simulink model "lateral_control"  (Simulink 7.6)
settings: Solver=FixedStepDiscrete  StartTime=0.0  StopTime=Tfin  FixedStep=Ts  RelTol=1e-3
undefined symbols (not defined in the file or in its folder): ailerons_max, ailerons_min, ailerons_trim, beta_trim, DiscIntNeverNeededParam, K_heading, K_roll, roll_trim, rollrate_trim, rudder_max, rudder_trim, yawrate_trim
libraries: simulink x2
settings Model: Creator=borjafons  LastModifiedBy=frafonal
settings OptimizationCC: InlineParams=on  OptimizeModelRefInitCode=on  LifeSpan=1
settings DebuggingCC: FcnCallInpInsideContextMsg=Enable All
settings RTWCC: SystemTargetFile=ert.tlc  GenCodeOnly=on  TemplateMakefile=ert_default_tmf  Description=Embedded Coder  ProcessScript=ert_make_rtw_hook
settings CodeAppCC: IgnoreCustomStorageClasses=off
settings ERTTargetCC: MultiwordLength=2048  GenerateSampleERTMain=on  SupportNonFinite=off  SupportComplex=off  InlinedParameterPlacement=NonHierarchical  ERTCustomFileTemplate=example_file_process.tlc  ConvertIfToSwitch=off

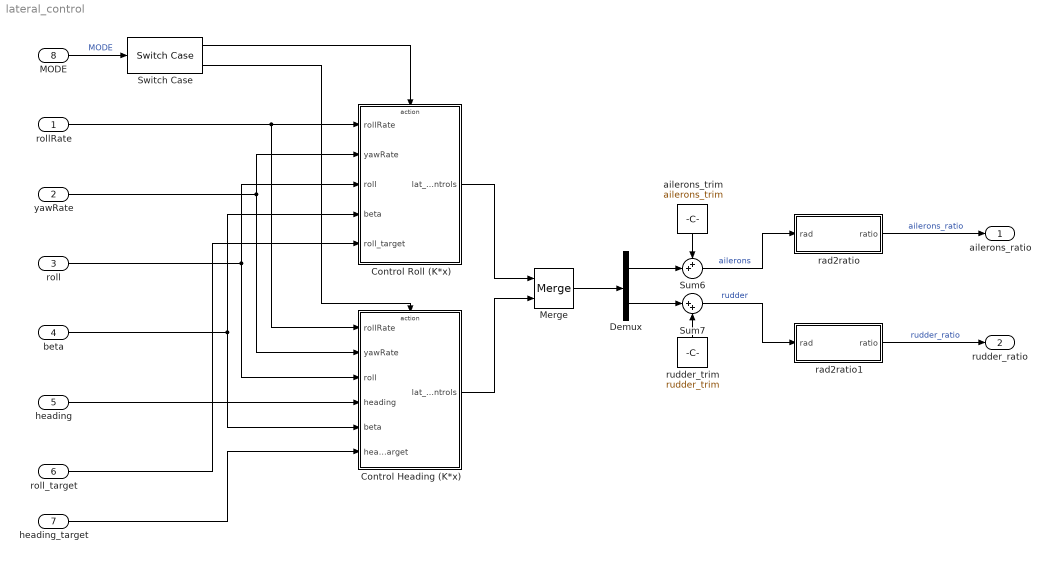
== system lateral_control ==
  rollRate : Inport
  yawRate : Inport  Port=2
  roll : Inport  Port=3
  beta : Inport  Port=4
  heading : Inport  Port=5
  roll_target : Inport  Port=6
  heading_target : Inport  Port=7
  MODE : Inport  Port=8
  Control Heading (K*x) : Subsystem  TreatAsAtomicUnit=on
  Control Roll (K*x) : Subsystem  TreatAsAtomicUnit=on
  Demux : Demux  Outputs=2
  Merge : Merge
  Sum6 : Sum  Inputs=++|
  Sum7 : Sum  Inputs=|++
  Switch Case : SwitchCase  CaseConditions={ROLL_CONTROL, HEADING_CONTROL}  ShowDefaultCase=off
  ailerons_trim : Constant  Value=ailerons_trim
  rad2ratio : Subsystem
  rad2ratio1 : Subsystem
  rudder_trim : Constant  Value=rudder_trim
  ailerons_ratio : Outport
  rudder_ratio : Outport  Port=2
  wires:
  Merge/1 -> Demux/1
  rad2ratio/1(ratio) -> ailerons_ratio/1  "ailerons_ratio"
  rad2ratio1/1(ratio) -> rudder_ratio/1  "rudder_ratio"
  ailerons_trim/1 -> Sum6/1
  Sum6/1 -> rad2ratio/1(rad)  "ailerons"
  Demux/1 -> Sum6/2
  rudder_trim/1 -> Sum7/2
  Demux/2 -> Sum7/1
  Sum7/1 -> rad2ratio1/1(rad)  "rudder"
  Control Roll (K*x)/1(lat_controls) -> Merge/1
  Control Heading (K*x)/1(lat_controls) -> Merge/2
  Switch Case/1 -> Control Roll (K*x)/Action
  MODE/1 -> Switch Case/1  "MODE"
  rollRate/1 -> Control Roll (K*x)/1(rollRate), Control Heading (K*x)/1(rollRate)
  yawRate/1 -> Control Roll (K*x)/2(yawRate), Control Heading (K*x)/2(yawRate)
  roll/1 -> Control Roll (K*x)/3(roll), Control Heading (K*x)/3(roll)
  beta/1 -> Control Roll (K*x)/4(beta), Control Heading (K*x)/5(beta)
  heading/1 -> Control Heading (K*x)/4(heading)
  roll_target/1 -> Control Roll (K*x)/5(roll_target)
  heading_target/1 -> Control Heading (K*x)/6(heading_target)
  Switch Case/2 -> Control Heading (K*x)/Action

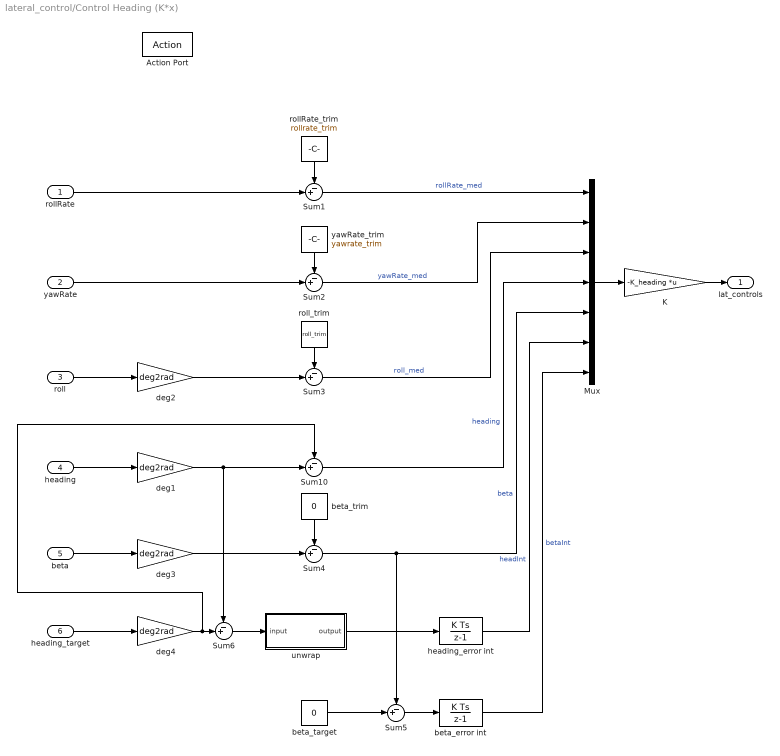
== system lateral_control/Control Heading (K*x) ==
  rollRate : Inport
  yawRate : Inport  Port=2
  roll : Inport  Port=3
  heading : Inport  Port=4
  beta : Inport  Port=5
  heading_target : Inport  Port=6
  Action Port : ActionPort  ActionType=case
  K : Gain  Gain=-K_heading  Multiplication=Matrix(K*u) (u vector)
  Mux : Mux  Inputs=7
  Sum{1..6,10} (7 alike) : Sum  Inputs=-+|
  beta_error int : DiscreteIntegrator  SampleTime=-1  LimitOutput=on  UpperSaturationLimit=5  LowerSaturationLimit=-5  ICPrevOutput=DiscIntNeverNeededParam  ICPrevScaledInput=DiscIntNeverNeededParam
  beta_target : Constant  Value=0
  beta_trim : Constant  Value=0
  deg{1..4} (4 alike) : Gain  Gain=deg2rad
  heading_error int : DiscreteIntegrator  SampleTime=-1  LimitOutput=on  UpperSaturationLimit=20  LowerSaturationLimit=-20  ICPrevOutput=DiscIntNeverNeededParam  ICPrevScaledInput=DiscIntNeverNeededParam
  rollRate_trim : Constant  Value=rollrate_trim
  roll_trim : Constant  Value=roll_trim
  unwrap : Subsystem
  yawRate_trim : Constant  Value=yawrate_trim
  lat_controls : Outport
  wires:
  Mux/1 -> K/1
  K/1 -> lat_controls/1
  rollRate_trim/1 -> Sum1/1
  rollRate/1 -> Sum1/2
  yawRate_trim/1 -> Sum2/1
  yawRate/1 -> Sum2/2
  roll_trim/1 -> Sum3/1
  roll/1 -> deg2/1
  deg2/1 -> Sum3/2
  Sum1/1 -> Mux/1  "rollRate_med"
  Sum2/1 -> Mux/2  "yawRate_med"
  Sum3/1 -> Mux/3  "roll_med"
  heading/1 -> deg1/1
  beta/1 -> deg3/1
  deg1/1 -> Sum10/2, Sum6/1
  beta_trim/1 -> Sum4/1
  deg3/1 -> Sum4/2
  Sum10/1 -> Mux/4  "heading"
  Sum4/1 -> Mux/5, Sum5/1  "beta"
  beta_target/1 -> Sum5/2
  Sum5/1 -> beta_error int/1
  beta_error int/1 -> Mux/7  "betaInt"
  heading_target/1 -> deg4/1
  deg4/1 -> Sum6/2, Sum10/1
  Sum6/1 -> unwrap/1(input)
  unwrap/1(output) -> heading_error int/1
  heading_error int/1 -> Mux/6  "headInt"

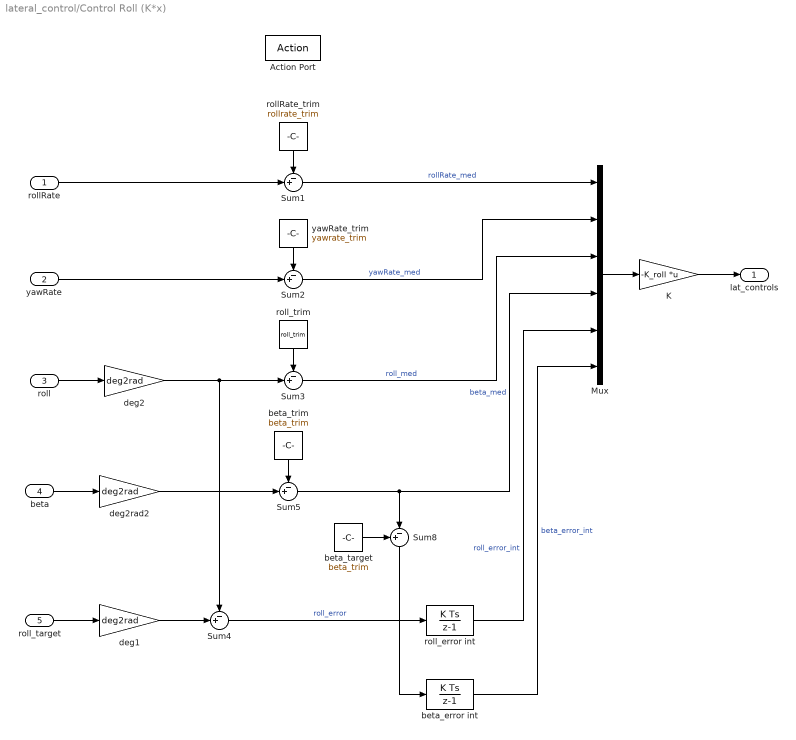
== system lateral_control/Control Roll (K*x) ==
  rollRate : Inport
  yawRate : Inport  Port=2
  roll : Inport  Port=3
  beta : Inport  Port=4
  roll_target : Inport  Port=5
  Action Port : ActionPort  ActionType=case
  K : Gain  Gain=-K_roll  Multiplication=Matrix(K*u) (u vector)
  Mux : Mux  Inputs=6
  Sum{1..5} (5 alike) : Sum  Inputs=-+|
  Sum8 : Sum  Inputs=+-|
  beta_error int : DiscreteIntegrator  SampleTime=-1  LimitOutput=on  UpperSaturationLimit=5  LowerSaturationLimit=-5  ICPrevOutput=DiscIntNeverNeededParam  ICPrevScaledInput=DiscIntNeverNeededParam
  beta_target : Constant  Value=beta_trim
  beta_trim : Constant  Value=beta_trim
  deg1 : Gain  Gain=deg2rad
  deg2 : Gain  Gain=deg2rad
  deg2rad2 : Gain  Gain=deg2rad
  rollRate_trim : Constant  Value=rollrate_trim
  roll_error int : DiscreteIntegrator  SampleTime=-1  LimitOutput=on  UpperSaturationLimit=8  LowerSaturationLimit=-8  ICPrevOutput=DiscIntNeverNeededParam  ICPrevScaledInput=DiscIntNeverNeededParam
  roll_trim : Constant  Value=roll_trim
  yawRate_trim : Constant  Value=yawrate_trim
  lat_controls : Outport
  wires:
  Mux/1 -> K/1
  K/1 -> lat_controls/1
  rollRate_trim/1 -> Sum1/1
  rollRate/1 -> Sum1/2
  yawRate_trim/1 -> Sum2/1
  yawRate/1 -> Sum2/2
  roll_trim/1 -> Sum3/1
  roll/1 -> deg2/1
  deg2/1 -> Sum3/2, Sum4/1
  beta_trim/1 -> Sum5/1
  deg2rad2/1 -> Sum5/2
  beta/1 -> deg2rad2/1
  Sum5/1 -> Sum8/2, Mux/4  "beta_med"
  roll_target/1 -> deg1/1
  Sum4/1 -> roll_error int/1  "roll_error"
  deg1/1 -> Sum4/2
  Sum8/1 -> beta_error int/1
  beta_target/1 -> Sum8/1
  Sum1/1 -> Mux/1  "rollRate_med"
  Sum2/1 -> Mux/2  "yawRate_med"
  Sum3/1 -> Mux/3  "roll_med"
  roll_error int/1 -> Mux/5  "roll_error_int"
  beta_error int/1 -> Mux/6  "beta_error_int"

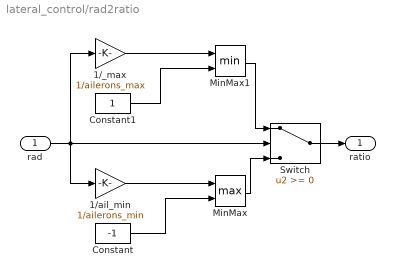
== system lateral_control/rad2ratio ==
  rad : Inport
  1/_max : Gain  Gain=1/ailerons_max
  1/ail_min : Gain  Gain=1/ailerons_min
  Constant : Constant  Value=-1
  Constant1 : Constant
  MinMax : MinMax  Function=max  Inputs=2
  MinMax1 : MinMax  Inputs=2
  Switch : Switch
  ratio : Outport
  wires:
  1/ail_min/1 -> MinMax/1
  Constant/1 -> MinMax/2
  MinMax/1 -> Switch/3
  1/_max/1 -> MinMax1/1
  Constant1/1 -> MinMax1/2
  MinMax1/1 -> Switch/1
  rad/1 -> Switch/2, 1/ail_min/1, 1/_max/1
  Switch/1 -> ratio/1

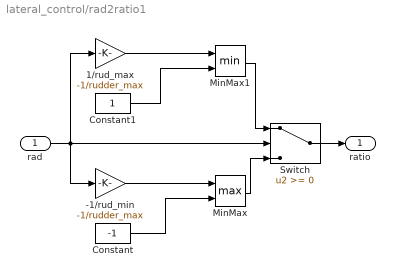
== system lateral_control/rad2ratio1 ==
  rad : Inport
  -1/rud_min : Gain  Gain=-1/rudder_max
  1/rud_max : Gain  Gain=-1/rudder_max
  Constant : Constant  Value=-1
  Constant1 : Constant
  MinMax : MinMax  Function=max  Inputs=2
  MinMax1 : MinMax  Inputs=2
  Switch : Switch
  ratio : Outport
  wires:
  Switch/1 -> ratio/1
  rad/1 -> 1/rud_max/1, -1/rud_min/1, Switch/2
  MinMax1/1 -> Switch/1
  Constant1/1 -> MinMax1/2
  1/rud_max/1 -> MinMax1/1
  MinMax/1 -> Switch/3
  Constant/1 -> MinMax/2
  -1/rud_min/1 -> MinMax/1

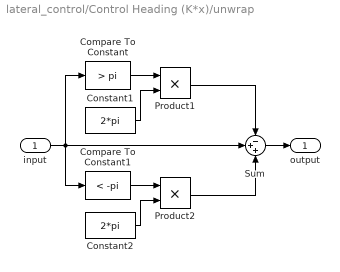
== system lateral_control/Control Heading (K*x)/unwrap ==
  input : Inport
  Compare To Constant : simulink/Logic and Bit Operations/Compare To Constant  SystemSampleTime=-1  relop=>  const=pi  LogicOutDataTypeMode=uint8
  Compare To Constant1 : simulink/Logic and Bit Operations/Compare To Constant  SystemSampleTime=-1  relop=<  const=-pi  LogicOutDataTypeMode=uint8
  Constant1 : Constant  Value=2*pi
  Constant2 : Constant  Value=2*pi
  Product1 : Product  RndMeth=Zero
  Product2 : Product  RndMeth=Zero
  Sum : Sum  Inputs=-++
  output : Outport
  wires:
  Compare To Constant/1 -> Product1/1
  Constant1/1 -> Product1/2
  Compare To Constant1/1 -> Product2/1
  Constant2/1 -> Product2/2
  Product1/1 -> Sum/1
  Product2/1 -> Sum/3
  Sum/1 -> output/1
  input/1 -> Sum/2, Compare To Constant/1, Compare To Constant1/1
